simulink model "mainDisPlantInversion"  (R2018b)
settings: Solver=VariableStepAuto  StartTime=0.0  StopTime=0.11  FixedStep=2e-4  RelTol=1e-3
values from neighbouring files (symbols this model uses):
  forwardOrder = numel(zero(delta))  - numel(pole(delta))    [calculateDelta.m]    (also in initSim.m = forwardOrderD + forwardOrderF; modelBasedFeedforward.m = numel(zero(feedforwardController)) - numel(pole(feedforwardC)
  Ts = 0.0002    [closedLoopIdentification.m]    (also in initSim.m; test.m)
libraries: cstblocks x3, model_controller x2
settings Model: Creator=Dai Luyao  LastModifiedBy=Princess
settings SFSimCC: SimUseLocalCustomCode=off
settings RTWCC: RTWUseLocalCustomCode=off
settings CodeAppCC: StateflowObjectComments=on

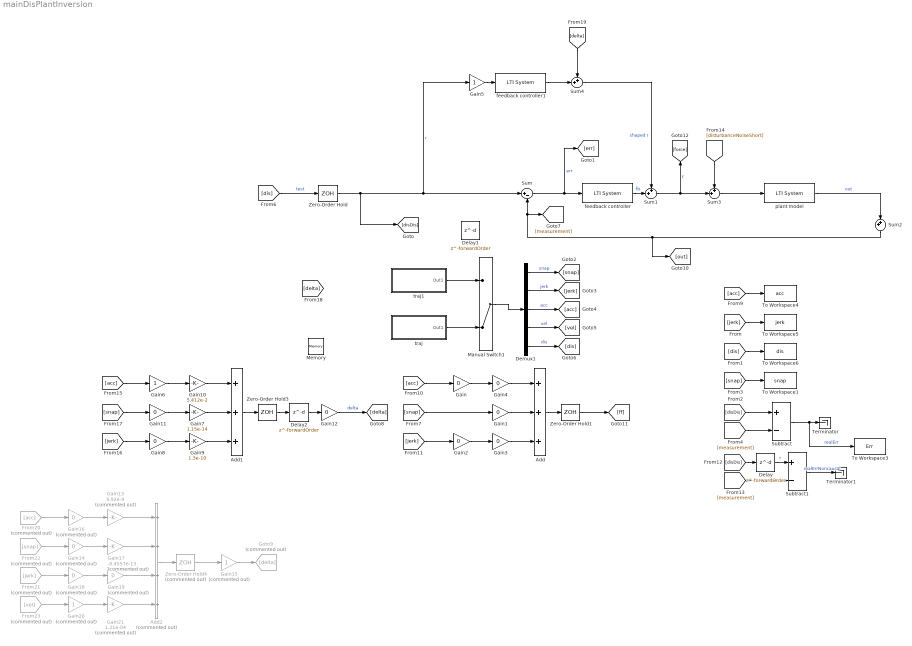
== system mainDisPlantInversion ==
  Add : Sum  Inputs=+++
  Add1 : Sum  Inputs=+++
  Add2 : Sum  Commented=on  Inputs=++++
  Delay : Delay  DelayLength=forwardOrder  SampleTime=Ts
  Delay1 : Delay  DelayLength=forwardOrder  SampleTime=Ts
  Delay2 : Delay  DelayLength=forwardOrder  SampleTime=Ts
  Demux1 : Demux  Outputs=5
  From20 : From  Commented=on  GotoTag=acc
  From21 : From  Commented=on  GotoTag=jerk
  From22 : From  Commented=on  GotoTag=snap
  From23 : From  Commented=on  GotoTag=vel
  Gain{,1..4,8,11..12} (8 alike) : Gain  Gain=0
  Gain10 : Gain  Gain=5.412e-2
  Gain13 : Gain  Commented=on  Gain=9.92e-9
  Gain{14,16,18..19} (4 alike) : Gain  Commented=on  Gain=0
  Gain15 : Gain  Commented=on
  Gain17 : Gain  Commented=on  Gain=-0.4557e-13
  Gain20 : Gain  Commented=on
  Gain21 : Gain  Commented=on  Gain=1.21e-04
  Gain5 : Gain
  Gain6 : Gain
  Gain7 : Gain  Gain=1.15e-14
  Gain9 : Gain  Gain=1.3e-10
  Goto9 : Goto  Commented=on  GotoTag=delta
  Manual Switch1 : ManualSwitch  CurrentSetting=0
  Memory : Memory
  Subtract : Sum  Inputs=+-
  Subtract1 : Sum  Inputs=+-
  Sum : Sum  Inputs=|+-
  Sum{1..4} (4 alike) : Sum  Inputs=++|
  Terminator : Terminator
  Terminator1 : Terminator
  To Workspace1 : ToWorkspace  VariableName=snap  SaveFormat=Structure With Time  SampleTime=-1
  To Workspace3 : ToWorkspace  VariableName=Err  SaveFormat=Structure With Time  SampleTime=-1
  To Workspace4 : ToWorkspace  VariableName=acc  SaveFormat=Structure With Time  SampleTime=-1
  To Workspace5 : ToWorkspace  VariableName=jerk  SaveFormat=Structure With Time  SampleTime=-1
  To Workspace6 : ToWorkspace  VariableName=dis  SaveFormat=Structure With Time  SampleTime=-1
  Zero-Order Hold : ZeroOrderHold  SampleTime=Ts
  Zero-Order Hold1 : ZeroOrderHold  SampleTime=Ts
  Zero-Order Hold3 : ZeroOrderHold  SampleTime=Ts
  Zero-Order Hold4 : ZeroOrderHold  Commented=on  SampleTime=Ts
  feedback controller : cstblocks/LTI System  sys=GcDis  IC=[]
  feedback controller1 : cstblocks/LTI System  sys=FCausal  IC=[]
  plant model : cstblocks/LTI System  sys=GpDis  IC=[]
  traj : Subsystem  BlockChoice=4th order traj
      link override 2nd order traj: Ts=Ts
      link override 3rd order traj: j=800  v=0.25  x=0.06  a=10
      link override 4th order traj: a=30  v=0.6  x=0.04  j=2000  d=1500000  Ts=Ts
      settings: AttributesFormatString=%<BlockChoice>  TemplateBlock=model_controller/Profile Generators/traj  MemberBlocks=2th order traj,3rd order traj,4th order traj,step
  traj1 : Subsystem  BlockChoice=4th order traj
      link override 3rd order traj: j=800  v=0.25  x=0.06  a=10
      link override 4th order traj: a=20  v=0.5  x=0.2  j=2000  d=1.5e6
      settings: AttributesFormatString=%<BlockChoice>  TemplateBlock=model_controller/Profile Generators/traj  MemberBlocks=2th order traj,3rd order traj,4th order traj,step
  wires:
  Sum/1 -> feedback controller/1, [err]  "err"
  feedback controller/1 -> Sum1/2  "fb"
  Sum1/1 -> Sum3/2, [force]  "f"
  plant model/1 -> Sum2/2  "out"
  Demux1/1 -> [snap]  "snap"
  Demux1/2 -> [jerk]  "jerk"
  Demux1/3 -> [acc]  "acc"
  Demux1/4 -> [vel]  "vel"
  Demux1/5 -> [dis]  "dis"
  [acc] -> To Workspace4/1
  [acc] -> Gain/1
  [jerk] -> To Workspace5/1
  [dis] -> To Workspace6/1
  [snap] -> To Workspace1/1
  [snap] -> Gain1/1
  Gain/1 -> Gain4/1
  Gain1/1 -> Add/2
  traj1/1(Out1) -> Manual Switch1/1
  traj/1(Out1) -> Manual Switch1/2
  Manual Switch1/1 -> Demux1/1
  Add/1 -> Zero-Order Hold1/1
  Zero-Order Hold1/1 -> [ff]
  Sum2/1 -> [out], Sum/2, [measurement]
  Gain2/1 -> Gain3/1
  [jerk] -> Gain2/1
  Gain3/1 -> Add/3
  Gain4/1 -> Add/1
  Sum3/1 -> plant model/1
  [disDis] -> Subtract/1
  [measurement] -> Subtract/2
  Subtract/1 -> To Workspace3/1, Terminator/1  "realErr"
  Subtract1/1 -> Terminator1/1  "realErrNoncausal"
  [measurement] -> Subtract1/2
  [disDis] -> Delay/1
  Delay/1 -> Subtract1/1  "r"
  [disturbanceNoiseShort] -> Sum3/1
  [dis] -> Zero-Order Hold/1  "test"
  Gain10/1 -> Add1/1
  Gain9/1 -> Add1/3
  [jerk] -> Gain8/1
  Gain8/1 -> Gain9/1
  Add1/1 -> Zero-Order Hold3/1
  Gain7/1 -> Add1/2
  Gain6/1 -> Gain10/1
  [snap] -> Gain11/1
  [acc] -> Gain6/1
  Gain11/1 -> Gain7/1
  Zero-Order Hold3/1 -> Delay2/1
  Gain12/1 -> [delta]  "delta"
  Gain19/1 -> Add2/3
  Gain14/1 -> Gain17/1
  From22/1 -> Gain14/1
  Add2/1 -> Zero-Order Hold4/1
  Gain18/1 -> Gain19/1
  Gain17/1 -> Add2/2
  From21/1 -> Gain18/1
  Zero-Order Hold4/1 -> Gain15/1
  From20/1 -> Gain16/1
  Gain15/1 -> Goto9/1
  Gain16/1 -> Gain13/1
  Gain13/1 -> Add2/1
  From23/1 -> Gain20/1
  Gain20/1 -> Gain21/1
  Gain21/1 -> Add2/4
  Delay2/1 -> Gain12/1
  Sum4/1 -> Sum1/1  "shaped r"
  Gain5/1 -> feedback controller1/1
  Zero-Order Hold/1 -> Sum/1, Gain5/1, [disDis]  "r"
  feedback controller1/1 -> Sum4/2
  [delta] -> Sum4/1

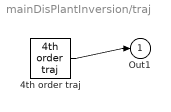
== system mainDisPlantInversion/traj ==
  4th order traj : model_controller/Profile Generators/4th order traj  t0=0  x=0.04  v=0.6  a=30  j=2000  d=1500000  Ts=Ts
  Out1 : Outport
  wires:
  4th order traj/1 -> Out1/1

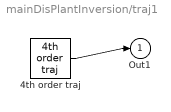
== system mainDisPlantInversion/traj1 ==
  4th order traj : model_controller/Profile Generators/4th order traj  t0=0  x=0.2  v=0.5  a=20  j=2000  d=1.5e6  Ts=0
  Out1 : Outport
  wires:
  4th order traj/1 -> Out1/1
